simulink model "sampleModel2032_sub_sub"  (R2023a)
settings: Solver=VariableStepAuto  StartTime=0.0  StopTime=10.0  RelTol=1e-3
libraries: hdlsllib x5, simulink x2
settings Model: Creator=user1  LastModifiedBy=user1
settings OptimizationCC: BlockReduction=off  ConditionallyExecuteInputs=off

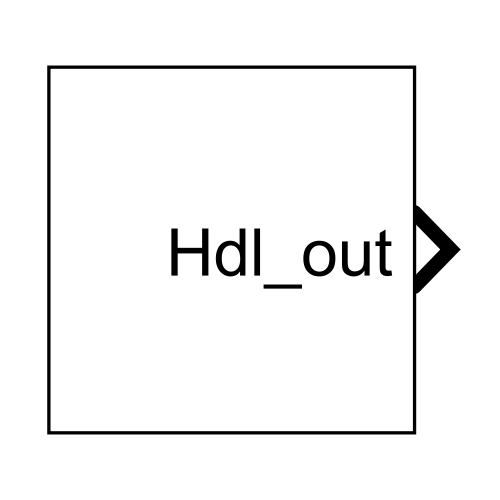
[thumbnail: Simulink's stored preview of the top-level diagram]
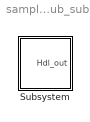
== system sampleModel2032_sub_sub ==
  Subsystem : Subsystem

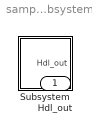
== system sampleModel2032_sub_sub/Subsystem ==
  Subsystem : Subsystem
  Hdl_out : Outport  OutDataTypeStr=uint8

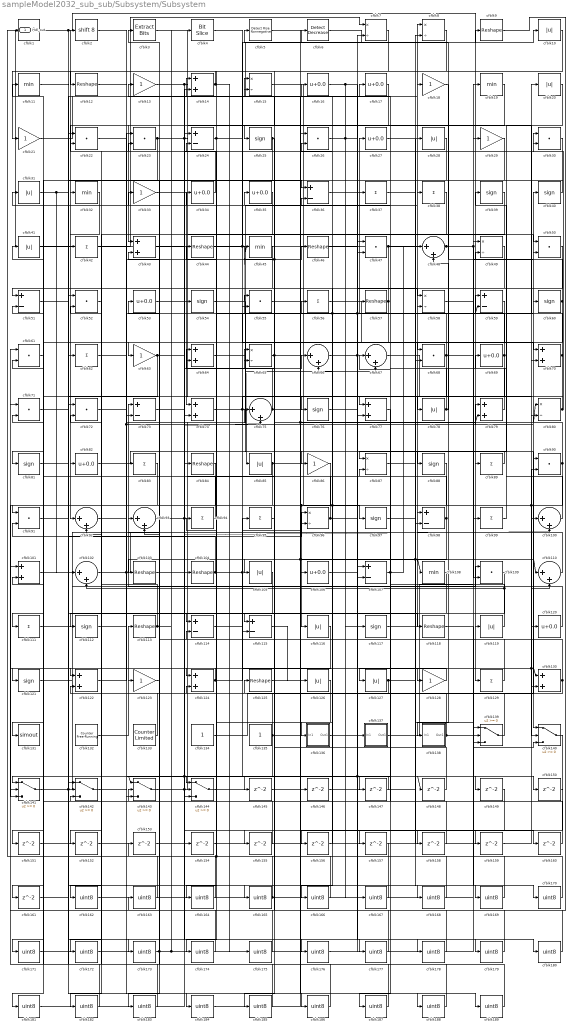
== system sampleModel2032_sub_sub/Subsystem/Subsystem ==
  cfblk1 : hdlsllib/Logic and Bit Operations/Compare To Zero  relop=<=  OutDataTypeStr=uint8
  cfblk{10,20,28,31,41,78,85,105,116,119,126..127} (12 alike) : Abs  OutDataTypeStr=uint8  SaturateOnIntegerOverflow=off
  cfblk{48,66..67,75,92..93,100,102,110} (9 alike) : Sum  Inputs=|++  OutDataTypeStr=uint8
  cfblk{14,43,64,70,74,77,79,101,122,124,130} (11 alike) : Sum  OutDataTypeStr=uint8
  cfblk{9,12,44,46,57,84,103..104,113,118,125} (11 alike) : Reshape
  cfblk{16..17,27,34..35,53,69,82,106,120} (10 alike) : Bias  Bias=0.0  SaturateOnIntegerOverflow=off
  cfblk{24,36,51,59,73,98,107,114..115} (9 alike) : Sum  Inputs=+-  OutDataTypeStr=uint8
  cfblk{11,19,32,45,108} (5 alike) : MinMax  OutDataTypeStr=uint8
  cfblk{22..23,26,30,47,50,52,55,61,68,71..72,90..91,109} (15 alike) : DotProduct  OutDataTypeStr=uint8
  cfblk{37..38,42,56,62,83,89,94..95,99,111,129} (12 alike) : Sum  Inputs=+  OutDataTypeStr=uint8
  cfblk{25,39..40,54,60,76,81,88,97,112,117,121} (12 alike) : Signum
  cfblk{13,18,21,29,33,63,86,123,128} (9 alike) : Gain  OutDataTypeStr=uint8
  cfblk131 : ToWorkspace  VariableName=simout  SaveFormat=Timeseries  SampleTime=-1
  cfblk132 : hdlsllib/Sources/Counter Free-Running  NumBits=16  tsamp=-1
  cfblk133 : hdlsllib/Sources/Counter Limited  uplimit=7  tsamp=-1
  cfblk134 : Constant  OutDataTypeStr=uint8  SampleTime=-1
  cfblk135 : Constant  OutDataTypeStr=uint8  SampleTime=-1
  cfblk136 : Subsystem
      settings: LibrarySourceBlock=|
      | hdlsllib/Ports &
      | Subsystems/Subsystem
  cfblk137 : Subsystem
      settings: LibrarySourceBlock=|
      | hdlsllib/Ports &
      | Subsystems/Subsystem
  cfblk138 : Subsystem
      settings: LibrarySourceBlock=|
      | hdlsllib/Ports &
      | Subsystems/Subsystem
  cfblk{139..144} (6 alike) : Switch  OutDataTypeStr=uint8  SaturateOnIntegerOverflow=off  InputSameDT=off
  cfblk{145..161} (17 alike) : Delay  SampleTime=1
  cfblk{7..8,15,49,58,65,80,87,96} (9 alike) : Product  Inputs=*/  OutDataTypeStr=uint8  RndMeth=Zero  SaturateOnIntegerOverflow=on
  cfblk{162..189} (28 alike) : DataTypeConversion  OutDataTypeStr=uint8  SaturateOnIntegerOverflow=off  RndMeth=Floor
  cfblk2 : ArithShift  BitShiftNumber=8
  cfblk3 : simulink/Logic and Bit Operations/Extract Bits  bitsToExtract=Upper half  numBits=8  bitIdxRange=[0 7]  outScalingMode=Preserve fixed-point scaling
      settings: LibrarySourceBlock=|
      | hdlsllib/Logic and Bit
      | Operations/Extract Bits
  cfblk4 : hdlsllib/Logic and Bit Operations/Bit Slice  lidx=7  ridx=0
  cfblk5 : hdlsllib/Logic and Bit Operations/Detect Rise Nonnegative  vinit=0  OutDataTypeStr=uint8
  cfblk6 : simulink/Logic and Bit Operations/Detect Decrease  vinit=0.0  OutDataTypeStr=uint8
      settings: LibrarySourceBlock=|
      | hdlsllib/Logic and Bit
      | Operations/Detect
      | Decrease
  Hdl_out : Outport  OutDataTypeStr=uint8
  wires:
  cfblk189/1 -> cfblk142/3
  cfblk188/1 -> cfblk142/2
  cfblk187/1 -> cfblk142/1
  cfblk150/1 -> cfblk187/1
  cfblk186/1 -> cfblk53/1
  cfblk142/1 -> cfblk186/1
  cfblk185/1 -> cfblk11/1
  cfblk184/1 -> cfblk26/1
  cfblk11/1 -> cfblk184/1
  cfblk183/1 -> cfblk61/2
  cfblk45/1 -> cfblk183/1
  cfblk182/1 -> cfblk61/1
  cfblk181/1 -> cfblk154/1
  cfblk61/1 -> cfblk181/1
  cfblk180/1 -> cfblk125/1
  cfblk179/1 -> cfblk35/1, cfblk45/1
  cfblk178/1 -> cfblk72/2
  cfblk177/1 -> cfblk72/1
  cfblk73/1 -> cfblk177/1
  cfblk176/1 -> cfblk139/1
  cfblk72/1 -> cfblk176/1
  cfblk175/1 -> cfblk101/2
  cfblk174/1 -> cfblk101/1
  cfblk126/1 -> cfblk174/1
  cfblk173/1 -> cfblk106/1, cfblk54/1, cfblk33/1
  cfblk172/1 -> cfblk84/1
  cfblk108/1 -> cfblk172/1
  cfblk171/1 -> cfblk47/1
  cfblk84/1 -> cfblk171/1
  cfblk170/1 -> cfblk71/2
  cfblk118/1 -> cfblk170/1
  cfblk169/1 -> cfblk71/1
  cfblk97/1 -> cfblk169/1
  cfblk168/1 -> cfblk64/2, cfblk24/1
  cfblk167/1 -> cfblk22/2
  cfblk166/1 -> cfblk22/1
  cfblk149/1 -> cfblk166/1
  cfblk165/1 -> cfblk153/1, cfblk29/1
  cfblk164/1 -> cfblk52/2
  cfblk105/1 -> cfblk164/1
  cfblk163/1 -> cfblk52/1
  cfblk9/1 -> cfblk163/1
  cfblk162/1 -> cfblk146/1
  cfblk52/1 -> cfblk162/1
  cfblk161/1 -> cfblk62/1
  cfblk83/1 -> cfblk161/1
  cfblk160/1 -> cfblk87/2
  cfblk43/1 -> cfblk160/1
  cfblk159/1 -> cfblk100/1
  cfblk158/1 -> cfblk51/2
  cfblk157/1 -> cfblk1/1
  cfblk77/1 -> cfblk157/1
  cfblk156/1 -> cfblk36/2
  cfblk155/1 -> cfblk93/2
  cfblk154/1 -> cfblk24/2
  cfblk153/1 -> cfblk90/2
  cfblk152/1 -> cfblk107/1
  cfblk38/1 -> cfblk152/1
  cfblk151/1 -> cfblk68/2
  cfblk53/1 -> cfblk150/1
  cfblk114/1 -> cfblk149/1
  cfblk148/1 -> cfblk15/2
  cfblk147/1 -> cfblk141/1
  cfblk109/1 -> cfblk147/1
  cfblk146/1 -> cfblk26/2
  cfblk145/1 -> cfblk98/2
  cfblk12/1 -> cfblk145/1
  cfblk26/1 -> cfblk80/2, cfblk167/1
  cfblk46/1 -> cfblk58/1
  cfblk101/1 -> cfblk173/1
  cfblk102/1 -> cfblk14/2, cfblk79/1
  cfblk140/1 -> cfblk143/2
  cfblk76/1 -> cfblk7/2
  cfblk13/1 -> cfblk120/1, cfblk100/2
  cfblk41/1 -> cfblk73/2
  cfblk99/1 -> cfblk39/1
  cfblk98/1 -> cfblk65/2, cfblk103/1
  cfblk94/1 -> cfblk23/2
  cfblk25/1 -> cfblk63/1, cfblk115/1
  cfblk49/1 -> cfblk66/2
  cfblk96/1 -> cfblk41/1, cfblk128/1
  cfblk24/1 -> cfblk144/1, cfblk10/1
  cfblk90/1 -> cfblk116/1, cfblk112/1, cfblk140/2, cfblk64/1
  cfblk123/1 -> cfblk43/2
  cfblk107/1 -> cfblk57/1, cfblk48/1
  cfblk4/1 -> cfblk70/1
  cfblk67/1 -> cfblk110/2
  cfblk59/1 -> cfblk91/1
  cfblk62/1 -> cfblk83/1
  cfblk113/1 -> cfblk92/2, cfblk4/1
  cfblk2/1 -> cfblk74/2
  cfblk23/1 -> cfblk50/1, cfblk155/1, cfblk143/3
  cfblk92/1 -> cfblk56/1
  cfblk89/1 -> cfblk87/1
  cfblk130/1 -> cfblk124/2, cfblk94/1
  cfblk135/1 -> cfblk143/1, cfblk144/3, cfblk17/1, cfblk79/2, cfblk114/2
  cfblk110/1 -> cfblk98/1
  cfblk36/1 -> cfblk68/1
  cfblk27/1 -> cfblk90/1
  cfblk71/1 -> cfblk168/1
  cfblk39/1 -> cfblk114/1
  cfblk122/1 -> cfblk46/1
  cfblk111/1 -> cfblk23/1
  cfblk82/1 -> cfblk86/1
  cfblk106/1 -> cfblk47/2, cfblk59/2
  cfblk60/1 -> cfblk5/1, cfblk151/1
  cfblk7/1 -> cfblk124/1
  cfblk144/1 -> cfblk37/1
  cfblk129/1 -> cfblk93/1
  cfblk19/1 -> cfblk43/1
  cfblk29/1 -> cfblk81/1
  cfblk6/1 -> cfblk9/1
  cfblk70/1 -> cfblk49/2, cfblk115/2
  cfblk35/1 -> cfblk55/2
  cfblk87/1 -> cfblk28/1
  cfblk132/1 -> cfblk123/1
  cfblk48/1 -> cfblk19/1, cfblk70/2, Hdl_out/1
  cfblk95/1 -> cfblk65/1
  cfblk31/1 -> cfblk36/1, cfblk102/1
  cfblk14/1 -> cfblk12/1, cfblk175/1
  cfblk16/1 -> cfblk117/1, cfblk158/1
  cfblk18/1 -> cfblk138/1(In1)
  cfblk28/1 -> cfblk107/2
  cfblk58/1 -> cfblk109/2
  cfblk104/1 -> cfblk130/1, cfblk130/2, cfblk95/1, cfblk91/2
  cfblk103/1 -> cfblk66/1
  cfblk65/1 -> cfblk185/1, cfblk188/1
  cfblk125/1 -> cfblk179/1
  cfblk127/1 -> cfblk122/2, cfblk60/1
  cfblk51/1 -> cfblk78/1
  cfblk75/1 -> cfblk88/1, cfblk34/1
  cfblk69/1 -> cfblk16/1, cfblk44/1, cfblk77/2
  cfblk93/1 -> cfblk20/1, cfblk75/2
  cfblk138/1(Out1) -> cfblk3/1, cfblk140/3
  cfblk88/1 -> cfblk141/3, cfblk156/1
  cfblk124/1 -> cfblk122/1, cfblk96/2
  cfblk81/1 -> cfblk14/1
  cfblk30/1 -> cfblk121/1
  cfblk63/1 -> cfblk104/1, cfblk131/1
  cfblk139/1 -> cfblk55/1
  cfblk3/1 -> cfblk137/1(In1)
  cfblk66/1 -> cfblk59/1, cfblk180/1
  cfblk116/1 -> cfblk141/2
  cfblk33/1 -> cfblk74/1
  cfblk10/1 -> cfblk25/1
  cfblk47/1 -> cfblk136/1(In1), cfblk139/3
  cfblk137/1(Out1) -> cfblk49/1
  cfblk141/1 -> cfblk8/2, cfblk96/1
  cfblk37/1 -> cfblk110/1, cfblk139/2
  cfblk100/1 -> cfblk69/1
  cfblk55/1 -> cfblk99/1
  cfblk86/1 -> cfblk111/1
  cfblk121/1 -> cfblk109/1
  cfblk34/1 -> cfblk2/1
  cfblk20/1 -> cfblk89/1
  cfblk79/1 -> cfblk13/1
  cfblk50/1 -> cfblk105/1
  cfblk64/1 -> cfblk67/2
  cfblk56/1 -> cfblk119/1
  cfblk136/1(Out1) -> cfblk148/1, cfblk178/1
  cfblk128/1 -> cfblk127/1
  cfblk74/1 -> cfblk38/1, cfblk58/2
  cfblk91/1 -> cfblk42/1
  cfblk22/1 -> cfblk165/1
  cfblk5/1 -> cfblk108/1, cfblk189/1
  cfblk119/1 -> cfblk67/1, cfblk102/2
  cfblk8/1 -> cfblk21/1
  cfblk57/1 -> cfblk51/1, cfblk144/2
  cfblk68/1 -> cfblk27/1, cfblk77/1, cfblk50/2
  cfblk112/1 -> cfblk80/1, cfblk75/1
  cfblk120/1 -> cfblk73/1
  cfblk117/1 -> cfblk8/1
  cfblk40/1 -> cfblk32/1
  cfblk80/1 -> cfblk76/1, cfblk30/1
  cfblk54/1 -> cfblk140/1
  cfblk17/1 -> cfblk82/1
  cfblk115/1 -> cfblk126/1
  cfblk78/1 -> cfblk31/1, cfblk48/2
  cfblk21/1 -> cfblk15/1
  cfblk1/1 -> cfblk129/1, cfblk118/1
  cfblk133/1 -> cfblk113/1
  cfblk42/1 -> cfblk7/1
  cfblk44/1 -> cfblk85/1, cfblk18/1
  cfblk143/1 -> cfblk6/1, cfblk30/2
  cfblk32/1 -> cfblk92/1
  cfblk15/1 -> cfblk97/1
  cfblk134/1 -> cfblk40/1
  cfblk85/1 -> cfblk159/1, cfblk182/1

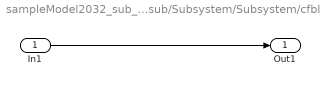
== system sampleModel2032_sub_sub/Subsystem/Subsystem/cfblk136 ==
  In1 : Inport
  Out1 : Outport
  wires:
  In1/1 -> Out1/1

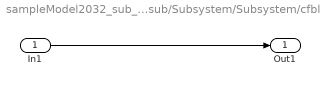
== system sampleModel2032_sub_sub/Subsystem/Subsystem/cfblk137 ==
  In1 : Inport
  Out1 : Outport
  wires:
  In1/1 -> Out1/1

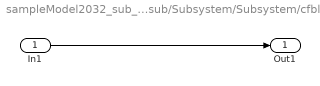
== system sampleModel2032_sub_sub/Subsystem/Subsystem/cfblk138 ==
  In1 : Inport
  Out1 : Outport
  wires:
  In1/1 -> Out1/1
